simulink subsystem "Sensors_SubSystem"  (R2020b)
settings: Solver=VariableStepAuto  StartTime=0.0  StopTime=10.0  RelTol=1e-3
settings Model: Creator=umberto  LastModifiedBy=Musta

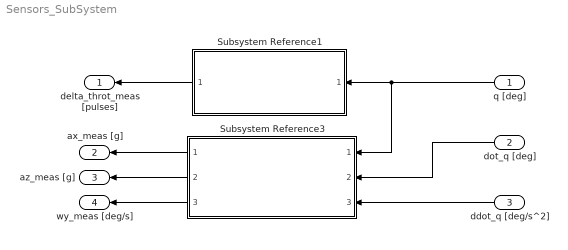
== system Sensors_SubSystem ==
  q [deg] : Inport
  dot_q [deg] : Inport  Port=2
  ddot_q [deg/s^2] : Inport  Port=3
  Subsystem Reference1 : Subsystem  ReferencedSubsystem=Encoder_SubSystem
  Subsystem Reference3 : Subsystem  ReferencedSubsystem=MPU_SubSystem
  delta_throt_meas [pulses] : Outport
  ax_meas [g] : Outport  Port=2
  az_meas [g] : Outport  Port=3
  wy_meas [deg/s] : Outport  Port=4
  wires:
  Subsystem Reference1/1 -> delta_throt_meas [pulses]/1
  Subsystem Reference3/2 -> az_meas [g]/1
  Subsystem Reference3/3 -> wy_meas [deg/s]/1
  Subsystem Reference3/1 -> ax_meas [g]/1
  q [deg]/1 -> Subsystem Reference3/1, Subsystem Reference1/1
  dot_q [deg]/1 -> Subsystem Reference3/2
  ddot_q [deg/s^2]/1 -> Subsystem Reference3/3
